simulink model "Inverted_pendulum_controller"  (R2019a)
settings: Solver=VariableStepAuto  StartTime=0.0  StopTime=10  RelTol=1e-3
values from neighbouring files (symbols this model uses):
  b = 0.05    [Inverted_pendulum_parameters.m]
  d = -0.005    [Inverted_pendulum_parameters.m]
  g = 9.81    [Inverted_pendulum_parameters.m]
  I = 0.099    [Inverted_pendulum_parameters.m]
  l = 0.4    [Inverted_pendulum_parameters.m]
  m = 0.23    [Inverted_pendulum_parameters.m]
  M = 2.4    [Inverted_pendulum_parameters.m]
libraries: simulink x2
settings Model: Creator=rajum  LastModifiedBy=rajum
settings DebuggingCC: UnconnectedInputMsg=none  UnconnectedOutputMsg=none  UnconnectedLineMsg=none
settings ModelReferenceCC: EnableRefExpFcnMdlSchedulingChecks=off
settings RTWCC: Description=Generic Real-Time Target

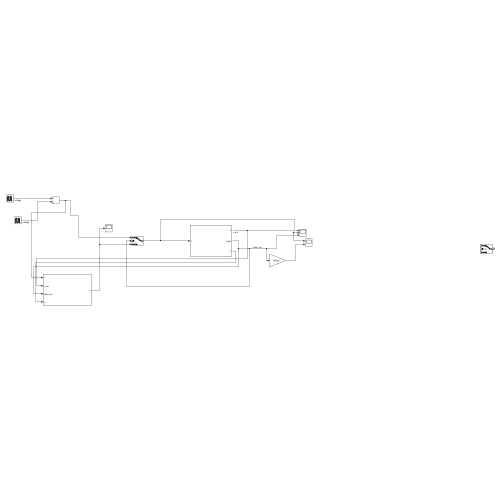
[thumbnail: Simulink's stored preview of the top-level diagram]
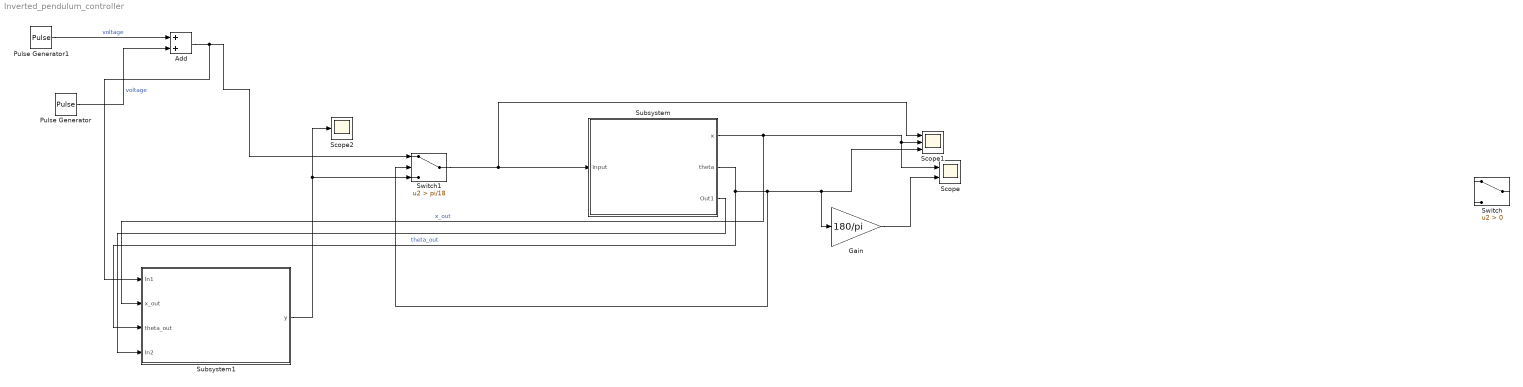
== system Inverted_pendulum_controller ==
  Add : Sum
  Gain : Gain  Gain=180/pi
  Pulse Generator : DiscretePulseGenerator  PulseType=Time based  Amplitude=14.5  Period=35  PulseWidth=0.1245  SampleTime=2
  Pulse Generator1 : DiscretePulseGenerator  PulseType=Time based  Amplitude=-14.5  Period=35  PulseWidth=0.1245  PhaseDelay=1.5  SampleTime=2
  Scope : Scope  NumInputPorts=2
  Scope1 : Scope  NumInputPorts=3
  Scope2 : Scope
  Subsystem : Subsystem
  Subsystem1 : Subsystem
  Switch : Switch  Criteria=u2 > Threshold
  Switch1 : Switch  Criteria=u2 > Threshold  Threshold=pi/18
  wires:
  Subsystem/2(theta) -> Subsystem1/3(theta_out), Switch1/2, Gain/1, Scope1/3  "theta_out"
  Subsystem/1(x) -> Subsystem1/2(x_out), Scope/1, Scope1/2  "x_out"
  Add/1 -> Subsystem1/1(In1), Switch1/1
  Pulse Generator1/1 -> Add/1  "voltage"
  Gain/1 -> Scope/2
  Switch1/1 -> Scope1/1, Subsystem/1(Input)
  Subsystem1/1(y) -> Scope2/1, Switch1/3
  Subsystem/3(Out1) -> Subsystem1/4(In2)
  Pulse Generator/1 -> Add/2  "voltage"

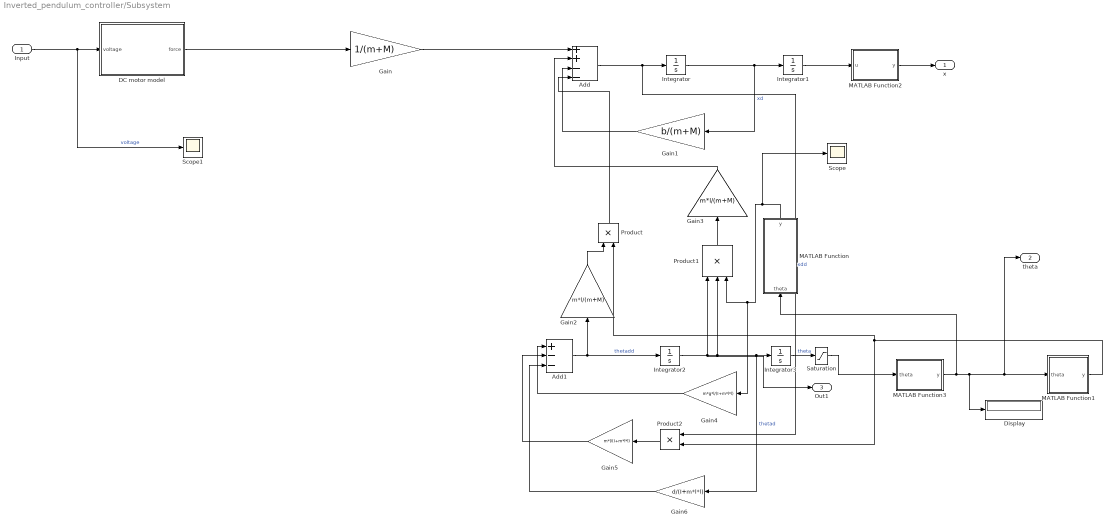
== system Inverted_pendulum_controller/Subsystem ==
  Input : Inport
  Add : Sum  Inputs=++--
  Add1 : Sum  Inputs=+--
  DC motor model : Subsystem
  Display : Display
  Gain : Gain  Gain=1/(m+M)
  Gain1 : Gain  Gain=b/(m+M)
  Gain2 : Gain  Gain=m*l/(m+M)
  Gain3 : Gain  Gain=m*l/(m+M)
  Gain4 : Gain  Gain=m*g*l/(I+m*l*l)
  Gain5 : Gain  Gain=m*l/(I+m*l*l)
  Gain6 : Gain  Gain=d/(I+m*l*l)
  Integrator : Integrator
  Integrator1 : Integrator
  Integrator2 : Integrator
  Integrator3 : Integrator  InitialCondition=pi
  MATLAB Function : MATLAB Function  TreatAsAtomicUnit=on
  MATLAB Function1 : MATLAB Function  TreatAsAtomicUnit=on
  MATLAB Function2 : MATLAB Function  TreatAsAtomicUnit=on
  MATLAB Function3 : MATLAB Function  TreatAsAtomicUnit=on
  Product : Product
  Product1 : Product  Inputs=3
  Product2 : Product
  Saturation : Saturate  UpperLimit=2*pi  LowerLimit=0
  Scope : Scope
  Scope1 : Scope
  x : Outport
  theta : Outport  Port=2
  Out1 : Outport  Port=3
  wires:
  Integrator3/1 -> Saturation/1  "theta"
  Add1/1 -> Integrator2/1, Gain2/1  "thetadd"
  Gain4/1 -> Add1/1
  Product1/1 -> Gain3/1
  Integrator/1 -> Gain1/1, Integrator1/1  "xd"
  Integrator2/1 -> Out1/1, Gain6/1, Integrator3/1, Product1/2, Product1/1  "thetad"
  Add/1 -> Product2/1, Integrator/1  "xdd"
  MATLAB Function1/1(y) -> Product/2, Product2/2
  MATLAB Function/1(y) -> Scope/1, Product1/3, Gain4/1
  Gain3/1 -> Add/2
  Product2/1 -> Gain5/1
  Gain1/1 -> Add/3
  Product/1 -> Add/4
  Integrator1/1 -> MATLAB Function2/1(u)
  Gain6/1 -> Add1/3
  Gain5/1 -> Add1/2
  DC motor model/1(force) -> Gain/1
  Gain/1 -> Add/1
  Gain2/1 -> Product/1
  MATLAB Function2/1(y) -> x/1
  Input/1 -> Scope1/1, DC motor model/1(voltage)  "voltage"
  Saturation/1 -> MATLAB Function3/1(theta)
  MATLAB Function3/1(y) -> Display/1, theta/1, MATLAB Function1/1(theta), MATLAB Function/1(theta)

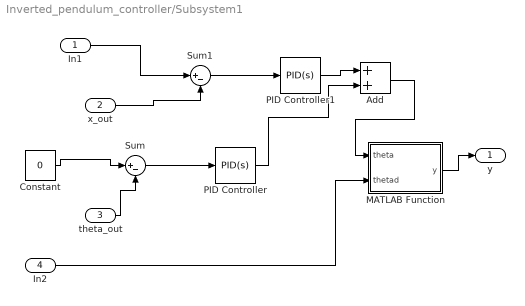
== system Inverted_pendulum_controller/Subsystem1 ==
  In1 : Inport
  x_out : Inport  Port=2
  theta_out : Inport  Port=3
  In2 : Inport  Port=4
  Add : Sum
  Constant : Constant  Value=0
  MATLAB Function : MATLAB Function  TreatAsAtomicUnit=on
  PID Controller : simulink/Continuous/PID Controller  Controller=PID  Form=Parallel  TimeDomain=Continuous-time  SampleTime=-1  IntegratorMethod=Forward Euler  FilterMethod=Forward Euler  ControllerParametersSource=internal  P=-100000  I=150  D=0.1  N=100  UseFilter=on  TunerSelectOption=Transfer Function Based (PID Tuner App)  InitialConditionSource=internal  InitialConditionForIntegrator=0  InitialConditionForFilter=0  DifferentiatorICPrevScaledInput=0  ExternalReset=none  TrackingMode=off  Kt=1  LimitOutput=off  UpperSaturationLimit=inf  LowerSaturationLimit=-inf  LinearizeAsGain=on  AntiWindupMode=none  Kb=1  POutMin=[]  POutMax=[]  IOutMin=[]  IOutMax=[]  DOutMin=[]  DOutMax=[]  NOutMin=[]  NOutMax=[]  SumOutMin=[]  SumOutMax=[]  SaturationOutMin=[]  SaturationOutMax=[]  PParamMin=[]  PParamMax=[]  IParamMin=[]  IParamMax=[]  DParamMin=[]  DParamMax=[]  NParamMin=[]  NParamMax=[]  KbParamMin=[]  KbParamMax=[]  KtParamMin=[]  KtParamMax=[]  KbOutMin=[]  KbOutMax=[]  KtOutMin=[]  KtOutMax=[]  IntegratorOutMin=[]  IntegratorOutMax=[]  FilterOutMin=[]  FilterOutMax=[]  SumI1OutMin=[]  SumI1OutMax=[]  SumI2OutMin=[]  SumI2OutMax=[]  SumI3OutMin=[]  SumI3OutMax=[]  SumI4OutMin=[]  SumI4OutMax=[]  SumDOutMin=[]  SumDOutMax=[]  DifferentiatorOutMin=[]  DifferentiatorOutMax=[]  FilterDiffOutCoefMin=[]  FilterDiffOutCoefMax=[]  ReciprocalOutMin=[]  ReciprocalOutMax=[]  SumDenOutMin=[]  SumDenOutMax=[]  SumNumOutMin=[]  SumNumOutMax=[]  DivideOutMin=[]  DivideOutMax=[]  IntegratorContinuousStateAttributes=''  IntegratorStateMustResolveToSignalObject=off  IntegratorRTWStateStorageClass=Auto  FilterContinuousStateAttributes=''  FilterStateMustResolveToSignalObject=off  FilterRTWStateStorageClass=Auto  ParallelPVariant=InternalParameters  IdealPVariant=Disabled  IVariant=InternalParameters  DVariant=InternalParameters  IntegratorVariant=Continuous  SatVariant=Disabled  AWVariant=Passthrough  PCopyVariant=Disabled  TRVariant=Disabled  FdbkBlocksVariant=Forward  IdealPFdbkVariant=Disabled  SatFdbkVariant=Disabled  DerivativeFilterVariant=ContFilter  NVariant=InternalParameters  NCopyVariant=Disabled  FilterICVariant=InternalICsFilter  IntegratorICVariant=InternalICs  ExternalResetVariant=Disabled  TRSumVariant=Passthrough  SumFdbkVariant=Disabled  SumVariant=Sum_PID
  PID Controller1 : simulink/Continuous/PID Controller  Controller=PID  Form=Parallel  TimeDomain=Continuous-time  SampleTime=-1  IntegratorMethod=Forward Euler  FilterMethod=Forward Euler  ControllerParametersSource=internal  P=10000  I=150  D=0.1  N=100  UseFilter=on  TunerSelectOption=Transfer Function Based (PID Tuner App)  InitialConditionSource=internal  InitialConditionForIntegrator=0  InitialConditionForFilter=0  DifferentiatorICPrevScaledInput=0  ExternalReset=none  TrackingMode=off  Kt=1  LimitOutput=off  UpperSaturationLimit=inf  LowerSaturationLimit=-inf  LinearizeAsGain=on  AntiWindupMode=none  Kb=1  POutMin=[]  POutMax=[]  IOutMin=[]  IOutMax=[]  DOutMin=[]  DOutMax=[]  NOutMin=[]  NOutMax=[]  SumOutMin=[]  SumOutMax=[]  SaturationOutMin=[]  SaturationOutMax=[]  PParamMin=[]  PParamMax=[]  IParamMin=[]  IParamMax=[]  DParamMin=[]  DParamMax=[]  NParamMin=[]  NParamMax=[]  KbParamMin=[]  KbParamMax=[]  KtParamMin=[]  KtParamMax=[]  KbOutMin=[]  KbOutMax=[]  KtOutMin=[]  KtOutMax=[]  IntegratorOutMin=[]  IntegratorOutMax=[]  FilterOutMin=[]  FilterOutMax=[]  SumI1OutMin=[]  SumI1OutMax=[]  SumI2OutMin=[]  SumI2OutMax=[]  SumI3OutMin=[]  SumI3OutMax=[]  SumI4OutMin=[]  SumI4OutMax=[]  SumDOutMin=[]  SumDOutMax=[]  DifferentiatorOutMin=[]  DifferentiatorOutMax=[]  FilterDiffOutCoefMin=[]  FilterDiffOutCoefMax=[]  ReciprocalOutMin=[]  ReciprocalOutMax=[]  SumDenOutMin=[]  SumDenOutMax=[]  SumNumOutMin=[]  SumNumOutMax=[]  DivideOutMin=[]  DivideOutMax=[]  IntegratorContinuousStateAttributes=''  IntegratorStateMustResolveToSignalObject=off  IntegratorRTWStateStorageClass=Auto  FilterContinuousStateAttributes=''  FilterStateMustResolveToSignalObject=off  FilterRTWStateStorageClass=Auto  ParallelPVariant=InternalParameters  IdealPVariant=Disabled  IVariant=InternalParameters  DVariant=InternalParameters  IntegratorVariant=Continuous  SatVariant=Disabled  AWVariant=Passthrough  PCopyVariant=Disabled  TRVariant=Disabled  FdbkBlocksVariant=Forward  IdealPFdbkVariant=Disabled  SatFdbkVariant=Disabled  DerivativeFilterVariant=ContFilter  NVariant=InternalParameters  NCopyVariant=Disabled  FilterICVariant=InternalICsFilter  IntegratorICVariant=InternalICs  ExternalResetVariant=Disabled  TRSumVariant=Passthrough  SumFdbkVariant=Disabled  SumVariant=Sum_PID
  Sum : Sum  Inputs=|+-
  Sum1 : Sum  Inputs=|+-
  y : Outport
  wires:
  Sum/1 -> PID Controller/1
  Constant/1 -> Sum/1
  theta_out/1 -> Sum/2
  MATLAB Function/1(y) -> y/1
  In2/1 -> MATLAB Function/2(thetad)
  x_out/1 -> Sum1/2
  Sum1/1 -> PID Controller1/1
  In1/1 -> Sum1/1
  PID Controller1/1 -> Add/1
  PID Controller/1 -> Add/2
  Add/1 -> MATLAB Function/1(theta)

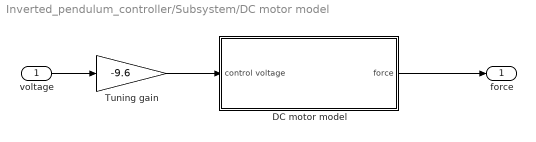
== system Inverted_pendulum_controller/Subsystem/DC motor model ==
  voltage : Inport
  DC motor model : Subsystem  mask{J=0.0000140, Kt=0.05, Kb=0.05, d=0.000001, R=2.5, L=0.0025}
      mask prompts: J "Moment of inertia"; Kt "Torque constant"; Kb "Electromotive force constant"; d "Linear approximation of viscous friction"; R "Electrical circuit resistance"; L "Electrical circuit inductance"
      mask Display: disp('DC motor')
  Tuning gain : Gain  Gain=-9.6
  force : Outport
  wires:
  Tuning gain/1 -> DC motor model/1(control voltage)
  voltage/1 -> Tuning gain/1
  DC motor model/1(force) -> force/1

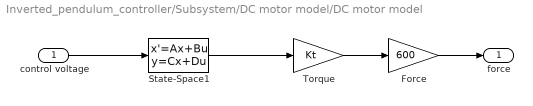
== system Inverted_pendulum_controller/Subsystem/DC motor model/DC motor model ==
  control voltage : Inport
  Force : Gain  Gain=600
  State-Space1 : StateSpace  A=[-d/J Kt/J;-Kb/L -R/L]  B=[0; 1/L]  C=[0 1]  D=0  InitialCondition=0
  Torque : Gain  Gain=Kt
  force : Outport
  wires:
  control voltage/1 -> State-Space1/1
  State-Space1/1 -> Torque/1
  Torque/1 -> Force/1
  Force/1 -> force/1

== matlab function Inverted_pendulum_controller/Subsystem/MATLAB Function2 ==
  data: u input; y output
function y = fcn(u)
if (u>0.3)
    y=0.3;
elseif (u<-0.3)
    y=-0.3;
else
    y = u;
end

== matlab function Inverted_pendulum_controller/Subsystem1/MATLAB Function ==
  data: theta input; y output; thetad input
function y = fcn(theta,thetad)
    if theta < 0.17453
        y = 0;
        thetad = 0;
    else
        y = theta;     
    end
end

== matlab function Inverted_pendulum_controller/Subsystem/MATLAB Function ==
  data: y output; theta input

function y = fcn(theta)
    if theta < 0.17453
        y = theta;
    else
        y = sin(theta);
    end
end

== matlab function Inverted_pendulum_controller/Subsystem/MATLAB Function1 ==
  data: theta input; y output

function y = fcn(theta)
    if theta < 0.17453
        y = 1;
    else
        y = cos(theta);
    end
end

== matlab function Inverted_pendulum_controller/Subsystem/MATLAB Function3 ==
  data: theta input; y output
function y = fcn(theta)
    if theta > 35*pi/180
        y = 2*pi - theta;
    else
        y = theta;
    end
end
